simulink model "PCS_3Phase_Grid"  (R2025a)
settings: Solver=ode4  StartTime=0.0  StopTime=0.5  FixedStep=1e-5  RelTol=1e-3
InitFcn:
  | v = str2double(get_param('PCS_3Phase_Grid/Vpcs_set', 'Value'));p = str2double(get_param('PCS_3Phase_Grid/Phase_set', 'Value'));set_param('PCS_3Phase_Grid/PCS', 'Voltage', num2str(v));set_param('PCS_3Phase_Grid/PCS', 'PhaseAngle', num2str(p));
libraries: spsThreePhaseSourceLib x2, spsThreePhaseSeriesRLCBranchLib x1, spsThreePhaseVIMeasurementLib x1, spspowerguiLib x1
Description:
  | Three-Phase PCS Simulation (native sps blocks)
  | R=0.1Ohm, L=5.0mH
  | P_total, Q_total = CONSTANT (no 100Hz ripple)
settings Model: Creator=jicai  LastModifiedBy=jicai

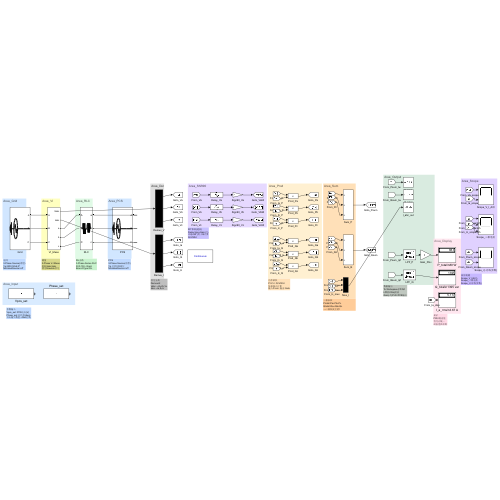
[thumbnail: Simulink's stored preview of the top-level diagram]
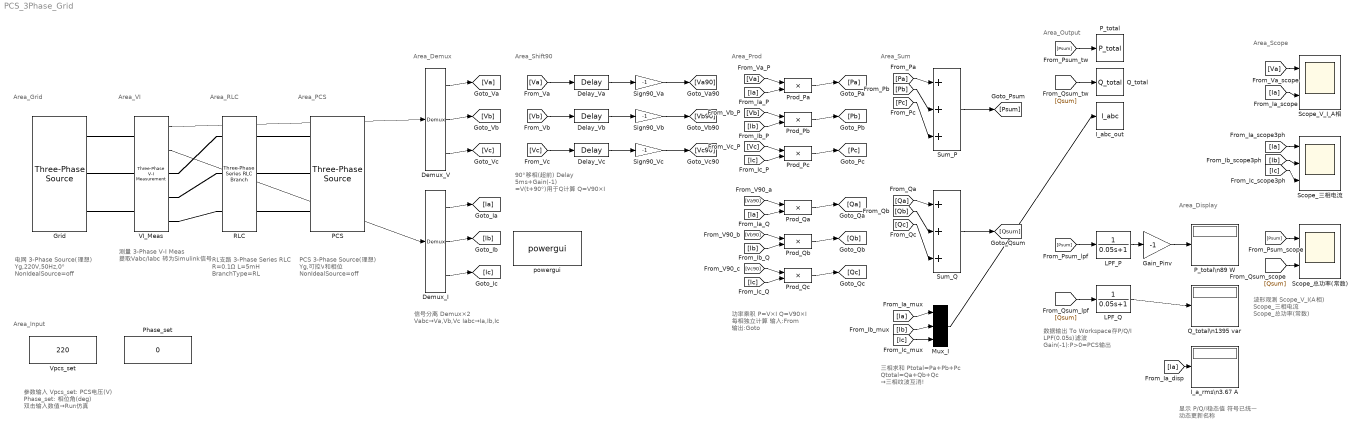
== system PCS_3Phase_Grid ==
  note: Area_Grid
  note: Area_VI
  note: Area_RLC
  note: Area_PCS
  note: Area_Demux
  note: Area_Shift90
  note: Area_Prod
  note: Area_Sum
  note: Area_Output
  note: Area_Display
  note: Area_Scope
  note: 电网
      | 3-Phase Source(理想)
      | Yg,220V,50Hz,0°
      | NonIdealSource=off
  note: RL支路
      | 3-Phase Series RLC
      | R=0.1Ω L=5mH
      | BranchType=RL
  note: 信号分离
      | Demux×2
      | Vabc→Va,Vb,Vc
      | Iabc→Ia,Ib,Ic
  note: 功率乘积
      | P=V×I  Q=V90×I
      | 每相独立计算
      | 输入:From  输出:Goto
  note: 显示
      | P/Q/I稳态值
      | 符号已统一
      | 动态更新名称
  note: 波形观测
      | Scope_V_I(A相)
      | Scope_三相电流
      | Scope_总功率(常数)
  note: 测量
      | 3-Phase V-I Meas
      | 提取Vabc/Iabc
      | 转为Simulink信号
  note: PCS
      | 3-Phase Source(理想)
      | Yg,可控V和相位
      | NonIdealSource=off
  note: 90°移相(超前)
      | Delay 5ms+Gain(-1)
      | =V(t+90°)用于Q计算
      | Q=V90×I
  note: 三相求和
      | Ptotal=Pa+Pb+Pc
      | Qtotal=Qa+Qb+Qc
      | →三相纹波互消!
  note: 数据输出
      | To Workspace存P/Q/I
      | LPF(0.05s)滤波
      | Gain(-1):P>0=PCS输出
  note: Area_Input
  note: 参数输入
      | Vpcs_set: PCS电压(V)
      | Phase_set: 相位角(deg)
      | 双击输入数值→Run仿真
  Delay_Va : TransportDelay  DelayTime=0.005
  Delay_Vb : TransportDelay  DelayTime=0.005
  Delay_Vc : TransportDelay  DelayTime=0.005
  Demux_I : Demux  Outputs=3
  Demux_V : Demux  Outputs=3
  Gain_Pinv : Gain  Gain=-1
  Grid : spsThreePhaseSourceLib/Three-Phase Source  InternalConnection=Yg  VoltagePhases=off  Voltage=220  PhaseAngle=0  Voltage_phases=[25e3 25e3 25e3]/sqrt(3)  PhaseAngles_phases=[0 -120 +120]  Frequency=50  NonIdealSource=off  SpecifyImpedance=off  Resistance=0.8929  Inductance=16.58e-3  ShortCircuitLevel=100e6  BaseVoltage=25e3  XRratio=7  BusType=swing  Pref=10e3  Qref=0  Prefabc=[10e3, 10e3, 10e3]  Qrefabc=[0, 0, 0]  Qmin=-inf  Qmax=inf
  I_a_rms\n3.67 A : Display
  I_abc_out : ToWorkspace  VariableName=I_abc  SampleTime=-1
  LPF_P : TransferFcn  Denominator=[0.05 1]
  LPF_Q : TransferFcn  Denominator=[0.05 1]
  Mux_I : Mux  Inputs=3
  PCS : spsThreePhaseSourceLib/Three-Phase Source  InternalConnection=Yg  VoltagePhases=off  Voltage=230  PhaseAngle=0  Voltage_phases=[25e3 25e3 25e3]/sqrt(3)  PhaseAngles_phases=[0 -120 +120]  Frequency=50  NonIdealSource=off  SpecifyImpedance=off  Resistance=0.8929  Inductance=16.58e-3  ShortCircuitLevel=100e6  BaseVoltage=25e3  XRratio=7  BusType=swing  Pref=10e3  Qref=0  Prefabc=[10e3, 10e3, 10e3]  Qrefabc=[0, 0, 0]  Qmin=-inf  Qmax=inf
  P_total : ToWorkspace  VariableName=P_total  SampleTime=-1
  P_total\n89 W : Display
  Phase_set : Constant  Value=0
  Prod_Pa : Product  Inputs=**
  Prod_Pb : Product  Inputs=**
  Prod_Pc : Product  Inputs=**
  Prod_Qa : Product  Inputs=**
  Prod_Qb : Product  Inputs=**
  Prod_Qc : Product  Inputs=**
  Q_total : ToWorkspace  VariableName=Q_total  SampleTime=-1
  Q_total\n1395 var : Display
  RLC : spsThreePhaseSeriesRLCBranchLib/Three-Phase Series RLC Branch  LConnTagsString=A|B|C  RConnTagsString=A|B|C  BranchType=RL  Resistance=0.1  Inductance=0.005  Capacitance=1e-6  Measurements=None
  Scope_V_I_A相 : Scope  NumInputPorts=2
  Scope_三相电流 : Scope  NumInputPorts=3
  Scope_总功率(常数) : Scope  NumInputPorts=2
  Sign90_Va : Gain  Gain=-1
  Sign90_Vb : Gain  Gain=-1
  Sign90_Vc : Gain  Gain=-1
  Sum_P : Sum  Inputs=+++
  Sum_Q : Sum  Inputs=+++
  VI_Meas : spsThreePhaseVIMeasurementLib/Three-Phase V-I Measurement  VoltageMeasurement=phase-to-ground  SetLabelV=off  LabelV=Vabc  Vpu=off  VpuLL=off  CurrentMeasurement=yes  SetLabelI=off  LabelI=Iabc  Ipu=off  Pbase=100e6  Vbase=500e3  OutputType=Complex  PhasorSimulation=off  PSBequivalent=0
  Vpcs_set : Constant  Value=220
  powergui : spspowerguiLib/powergui  Priority=1  SimulationMode=Continuous  SampleTime=50e-6  frequency=60  Iterations=50  frequencyindice=50  Pbase=100e6  ErrMax=1e-4  UnitsV=kV  UnitsW=MW  buscounter=0  FunctionMessages=off  echomessages=off  EnableUseOfTLC=off  CurrentSourceSwitches=off  DisableSnubberDevices=off  DisableRonSwitches=off  DisableVfSwitches=off  DisplayEquations=off  AutomaticDiscreteSolvers=off  SolverType=Tustin/Backward Euler (TBE)  Interpol=off  ExternalGateDelay=off  methode=off  Ts=100  x0status=blocks  SPID=on  SwTol=0  HookPort=off  NonlinearTolerance=1e-4  nMaxIteration=100  ContinueOnMaxIteration=off  RestoreLinks=warning  ResistiveCurrentMeasurement=off  Frange=[0:2:500]  Ylog=off  Xlog=on  ShowGrid=off  save=off  variable=ZData  structure=0  ZoomFFT=off  StartTime=0.0  cycles=1  DisplayStyle=1  fundamental=60  FreqAxis=off  MaxFrequency=1000  frequencyindicesteady=1  RmsSteady=1  display=off
  wires:
  VI_Meas/1 -> Demux_V/1
  VI_Meas/2 -> Demux_I/1
  Demux_V/1 -> [Va]
  Demux_I/1 -> [Ia]
  Demux_V/2 -> [Vb]
  Demux_I/2 -> [Ib]
  Demux_V/3 -> [Vc]
  Demux_I/3 -> [Ic]
  [Va] -> Delay_Va/1
  Delay_Va/1 -> Sign90_Va/1
  Sign90_Va/1 -> [Va90]
  [Vb] -> Delay_Vb/1
  Delay_Vb/1 -> Sign90_Vb/1
  Sign90_Vb/1 -> [Vb90]
  [Vc] -> Delay_Vc/1
  Delay_Vc/1 -> Sign90_Vc/1
  Sign90_Vc/1 -> [Vc90]
  [Va] -> Prod_Pa/1
  [Ia] -> Prod_Pa/2
  Prod_Pa/1 -> [Pa]
  [Va90] -> Prod_Qa/1
  [Ia] -> Prod_Qa/2
  Prod_Qa/1 -> [Qa]
  [Vb] -> Prod_Pb/1
  [Ib] -> Prod_Pb/2
  Prod_Pb/1 -> [Pb]
  [Vb90] -> Prod_Qb/1
  [Ib] -> Prod_Qb/2
  Prod_Qb/1 -> [Qb]
  [Vc] -> Prod_Pc/1
  [Ic] -> Prod_Pc/2
  Prod_Pc/1 -> [Pc]
  [Vc90] -> Prod_Qc/1
  [Ic] -> Prod_Qc/2
  Prod_Qc/1 -> [Qc]
  [Pa] -> Sum_P/1
  [Qa] -> Sum_Q/1
  [Pb] -> Sum_P/2
  [Qb] -> Sum_Q/2
  [Pc] -> Sum_P/3
  [Qc] -> Sum_Q/3
  Sum_P/1 -> [Psum]
  Sum_Q/1 -> [Qsum]
  [Ia] -> Mux_I/1
  [Ib] -> Mux_I/2
  [Ic] -> Mux_I/3
  [Psum] -> P_total/1
  [Qsum] -> Q_total/1
  Mux_I/1 -> I_abc_out/1
  [Psum] -> LPF_P/1
  [Qsum] -> LPF_Q/1
  LPF_P/1 -> Gain_Pinv/1
  Gain_Pinv/1 -> P_total\n89 W/1
  LPF_Q/1 -> Q_total\n1395 var/1
  [Ia] -> I_a_rms\n3.67 A/1
  [Va] -> Scope_V_I_A相/1
  [Ia] -> Scope_V_I_A相/2
  [Ia] -> Scope_三相电流/1
  [Ib] -> Scope_三相电流/2
  [Ic] -> Scope_三相电流/3
  [Psum] -> Scope_总功率(常数)/1
  [Qsum] -> Scope_总功率(常数)/2
  connections:
  Grid/RConn1 -- VI_Meas/LConn1
  VI_Meas/RConn1 -- RLC/LConn1
  RLC/RConn1 -- PCS/RConn1
  Grid/RConn2 -- VI_Meas/LConn2
  VI_Meas/RConn2 -- RLC/LConn2
  RLC/RConn2 -- PCS/RConn2
  Grid/RConn3 -- VI_Meas/LConn3
  VI_Meas/RConn3 -- RLC/LConn3
  RLC/RConn3 -- PCS/RConn3
